simulink model "hw6_1_5"  (R2013a)
settings: Solver=VariableStepDiscrete  StartTime=0.0  StopTime=30.0  RelTol=1e-3
libraries: dspsrcs4 x1
settings Model: Creator=cory  LastModifiedBy=cory

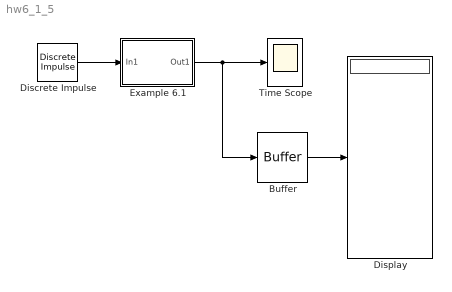
== system hw6_1_5 ==
  Buffer : Buffer  N=10
  Discrete Impulse : dspsrcs4/Discrete  Impulse  Delay=0  SampleTime=1  FrameSample=1  dataType=double  isSigned=on  wordLen=16  udDataType=sfix(16)  fracBitsMode=Best precision  numFracBits=15  OutDataTypeStr=double  LastOutDataTypeStr=double
  Display : Display
  Example 6.1 : Subsystem
  Time Scope : Scope
      settings: DataFormat=Structure
  wires:
  Example 6.1/1(Out1) -> Time Scope/1, Buffer/1
  Discrete Impulse/1 -> Example 6.1/1(In1)
  Buffer/1 -> Display/1

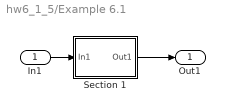
== system hw6_1_5/Example 6.1 ==
  In1 : Inport
  Section 1 : Subsystem
  Out1 : Outport
  wires:
  Section 1/1(Out1) -> Out1/1
  In1/1 -> Section 1/1(In1)

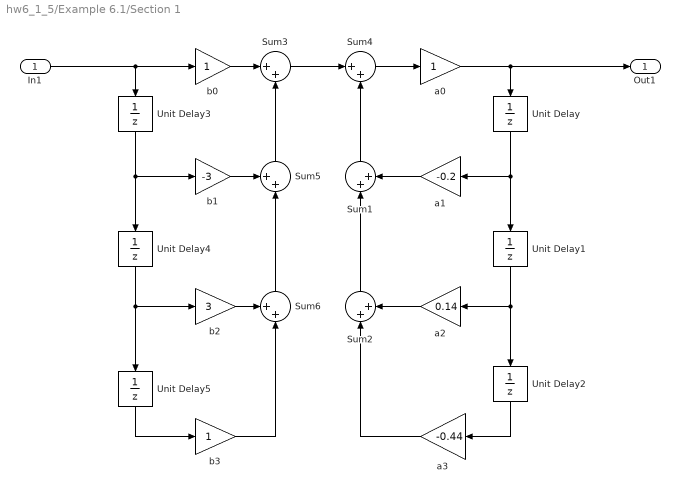
== system hw6_1_5/Example 6.1/Section 1 ==
  In1 : Inport
  Sum{1..4} (4 alike) : Sum  Inputs=|++
  Sum5 : Sum  Inputs=++|
  Sum6 : Sum  Inputs=++|
  Unit Delay{,1..5} (6 alike) : UnitDelay  SampleTime=-1
  a0 : Gain
  a1 : Gain  Gain=-0.2
  a2 : Gain  Gain=0.14
  a3 : Gain  Gain=-0.44
  b0 : Gain
  b1 : Gain  Gain=-3
  b2 : Gain  Gain=3
  b3 : Gain
  Out1 : Outport
  wires:
  a0/1 -> Out1/1, Unit Delay/1
  Sum4/1 -> a0/1
  Unit Delay/1 -> Unit Delay1/1, a1/1
  Unit Delay1/1 -> Unit Delay2/1, a2/1
  a1/1 -> Sum1/2
  Sum1/1 -> Sum4/2
  a2/1 -> Sum2/2
  Sum2/1 -> Sum1/1
  Unit Delay2/1 -> a3/1
  a3/1 -> Sum2/1
  In1/1 -> Unit Delay3/1, b0/1
  b0/1 -> Sum3/1
  Unit Delay3/1 -> Unit Delay4/1, b1/1
  b1/1 -> Sum5/1
  Sum5/1 -> Sum3/2
  Sum3/1 -> Sum4/1
  Unit Delay4/1 -> b2/1, Unit Delay5/1
  b3/1 -> Sum6/2
  Unit Delay5/1 -> b3/1
  b2/1 -> Sum6/1
  Sum6/1 -> Sum5/2
